simulink model "gm_sampleModel1782_4_sub"  (R2023a)
settings: Solver=VariableStepAuto  StartTime=0.0  StopTime=10.0  RelTol=1e-3
libraries: hdlsllib x1
settings Model: Creator=user1  LastModifiedBy=user1
settings OptimizationCC: BlockReduction=off  ConditionallyExecuteInputs=off
settings DebuggingCC: InheritedTsInSrcMsg=none

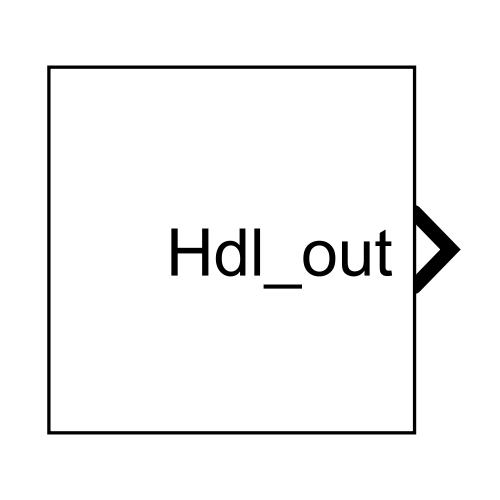
[thumbnail: Simulink's stored preview of the top-level diagram]
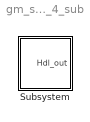
== system gm_sampleModel1782_4_sub ==
  Subsystem : Subsystem

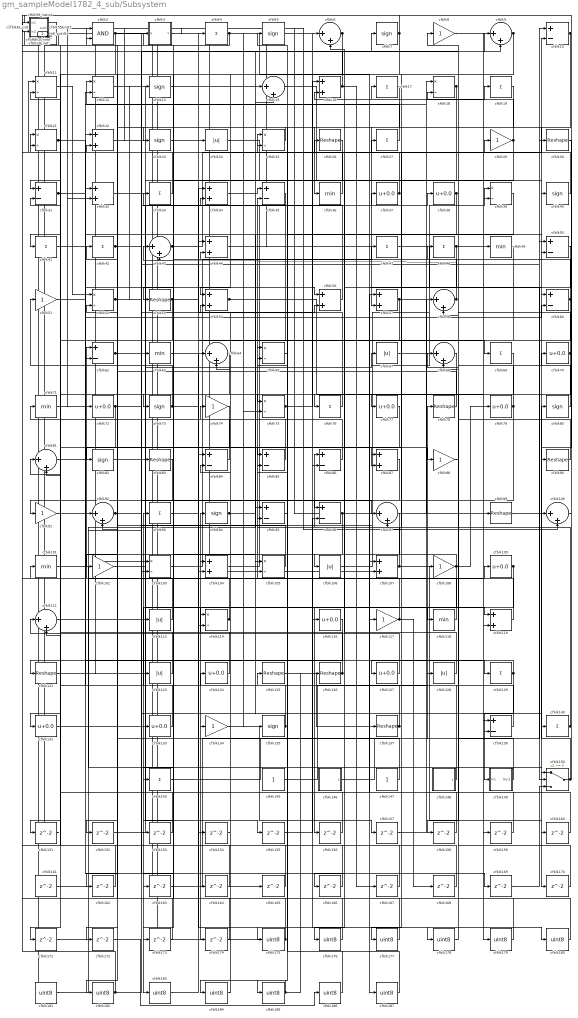
== system gm_sampleModel1782_4_sub/Subsystem ==
  cfblk1 : hdlsllib/Logic and Bit Operations/Bit Slice  lidx=7  ridx=0
  cfblk{10,31,35,50,60,62,84..86,95..96,139} (12 alike) : Sum  Inputs=+-  OutDataTypeStr=uint8
  cfblk{6,9,15,43,58,64,68,81,92,97,100,111} (12 alike) : Sum  Inputs=|++  OutDataTypeStr=uint8
  cfblk{36,49,63,71,101,118} (6 alike) : MinMax  OutDataTypeStr=uint8
  cfblk{8,29,51,74,88,91,102,108,117,134} (10 alike) : Gain  OutDataTypeStr=uint8
  cfblk{11..12,18,21,25,39,52,65,75,103,105,114} (12 alike) : Product  Inputs=*/  OutDataTypeStr=uint8  RndMeth=Zero  SaturateOnIntegerOverflow=on
  cfblk{16,22,32,34,44,54,56..57,87,104,107,119} (12 alike) : Sum  OutDataTypeStr=uint8
  cfblk{24,67,106,113,123,128} (6 alike) : Abs  OutDataTypeStr=uint8  SaturateOnIntegerOverflow=off
  cfblk{37..38,70,72,77,79,109,116,124,127,131,133} (12 alike) : Bias  Bias=0.0  SaturateOnIntegerOverflow=off
  cfblk110_inst : Subsystem
  cfblk112_inst : Subsystem
  cfblk115_inst : Subsystem
  cfblk{26,30,53,78,83,90,99,121,125..126,137} (11 alike) : Reshape
  cfblk122_inst : Subsystem
  cfblk{4,17,19,27,33,41..42,47..48,69,76,93,129,140,143} (15 alike) : Sum  Inputs=+  OutDataTypeStr=uint8
  cfblk{5,7,13,23,40,73,80,82,94,135} (10 alike) : Signum
  cfblk136_inst : Subsystem
  cfblk138_inst : Subsystem
  cfblk145 : Constant  OutDataTypeStr=uint8  SampleTime=-1
  cfblk146 : Subsystem  mask(Counter Limited){uplimit=double(7), tsamp=double(-1)}
      mask prompts: uplimit "Simulink:masks:UpperLimit_MP"; tsamp "Simulink:masks:SampleTime_MP"
      mask help: Simulink:masks:CounterLimited_MD
      mask init:
      | nbits = double(8);
      | tsamp = double(-1);
      | uplimit = double(7);
  cfblk147 : Constant  OutDataTypeStr=uint8  SampleTime=-1
  cfblk148 : Subsystem  mask(Counter Limited){uplimit=double(7), tsamp=double(-1)}
      mask prompts: uplimit "Simulink:masks:UpperLimit_MP"; tsamp "Simulink:masks:SampleTime_MP"
      mask help: Simulink:masks:CounterLimited_MD
      mask init:
      | nbits = double(8);
      | tsamp = double(-1);
      | uplimit = double(7);
  cfblk149 : Subsystem
  cfblk14_inst : Subsystem
  cfblk150 : Switch  OutDataTypeStr=uint8  SaturateOnIntegerOverflow=off  InputSameDT=off
  cfblk{151..174} (24 alike) : Delay  SampleTime=1
  cfblk{175..187} (13 alike) : DataTypeConversion  OutDataTypeStr=uint8  SaturateOnIntegerOverflow=off  RndMeth=Floor
  cfblk2 : Logic  AllPortsSameDT=off  OutDataTypeStr=boolean
  cfblk20_inst : Subsystem
  cfblk28_inst : Subsystem
  cfblk3 : Subsystem  mask(Detect Fall Nonpositive){vinit=double(0), InputProcessing=Elements as channels (sample based), OutDataTypeStr=uint8}
      mask prompts: vinit "Simulink:masks:InitialCondition_MP"; InputProcessing "Simulink:masks:InputProcessing_MP"; OutDataTypeStr "Simulink:masks:OutputDataType_MP"
      mask help: Simulink:masks:DetectFallNonpositive_MD
      mask init:
      | InputProcessing = 'Elements as channels (sample based)';
      | OutDataTypeStr = 'uint8';
      | vinit = double(0);
      mask TypeOptions InputProcessing: Simulink:masks:ColumnsAsChannelsFrameBased | Simulink:masks:ElementsAsChannelsSampleBased
      mask TypeOptions OutDataTypeStr: Simulink:masks:uint8 | Simulink:masks:boolean
      mask Display: fprintf('U <= 0\n&  NOT\nU/z <= 0')
  cfblk55_inst : Subsystem
  cfblk59_inst : Subsystem
  cfblk61_inst : Subsystem
  Hdl_out : Outport  OutDataTypeStr=uint8  SampleTime=1
  wires:
  cfblk1/1 -> cfblk61_inst/2(in2)
  cfblk10/1 -> cfblk57/2, cfblk170/1, cfblk36/1
  cfblk100/1 -> cfblk115_inst/1(in1)
  cfblk101/1 -> cfblk150/1
  cfblk102/1 -> cfblk119/1
  cfblk103/1 -> cfblk47/1
  cfblk104/1 -> cfblk37/1
  cfblk105/1 -> cfblk122_inst/2(in2)
  cfblk106/1 -> cfblk39/1
  cfblk107/1 -> cfblk35/2, cfblk160/1
  cfblk108/1 -> cfblk79/1, cfblk183/1, cfblk106/1, cfblk174/1
  cfblk109/1 -> cfblk156/1, cfblk134/1
  cfblk11/1 -> cfblk52/1
  cfblk110_inst/1(out1) -> cfblk32/2
  cfblk111/1 -> cfblk67/1
  cfblk112_inst/1(out1) -> cfblk6/1
  cfblk113/1 -> cfblk42/1
  cfblk114/1 -> cfblk62/1, cfblk138_inst/1(in1)
  cfblk115_inst/1(out1) -> cfblk24/1, cfblk14_inst/1(in1)
  cfblk116/1 -> cfblk121/1
  cfblk117/1 -> cfblk2/1, cfblk168/1
  cfblk118/1 -> cfblk95/2
  cfblk119/1 -> cfblk92/1
  cfblk12/1 -> cfblk155/1
  cfblk121/1 -> cfblk109/1
  cfblk122_inst/1(out1) -> cfblk20_inst/2(in2)
  cfblk123/1 -> cfblk28_inst/1(in1)
  cfblk124/1 -> cfblk59_inst/1(in1)
  cfblk125/1 -> cfblk137/1
  cfblk126/1 -> cfblk94/1, cfblk110_inst/2(in2)
  cfblk127/1 -> cfblk111/1
  cfblk128/1 -> cfblk6/2
  cfblk129/1 -> cfblk127/1, cfblk149/1(In1)
  cfblk13/1 -> cfblk15/1
  cfblk131/1 -> cfblk38/1
  cfblk133/1 -> cfblk101/1
  cfblk134/1 -> cfblk157/1
  cfblk135/1 -> cfblk125/1, cfblk21/1
  cfblk136_inst/1(out1) -> cfblk49/1
  cfblk137/1 -> cfblk21/2, cfblk93/1
  cfblk138_inst/1(out1) -> cfblk14_inst/2(in2), cfblk4/1
  cfblk139/1 -> cfblk74/1
  cfblk14_inst/1(out1) -> cfblk107/2, cfblk161/1
  cfblk140/1 -> cfblk86/1, cfblk27/1
  cfblk143/1 -> cfblk107/1
  cfblk145/1 -> cfblk78/1
  cfblk146/1(y) -> cfblk128/1
  cfblk147/1 -> cfblk62/2
  cfblk148/1(y) -> cfblk32/1
  cfblk149/1(Out1) -> cfblk108/1
  cfblk15/1 -> cfblk119/2
  cfblk150/1 -> cfblk80/1, cfblk70/1
  cfblk151/1 -> cfblk1/1
  cfblk152/1 -> cfblk39/2
  cfblk153/1 -> cfblk22/2
  cfblk154/1 -> cfblk84/2
  cfblk155/1 -> cfblk96/2
  cfblk156/1 -> cfblk85/2
  cfblk157/1 -> cfblk58/1
  cfblk158/1 -> cfblk81/1
  cfblk159/1 -> cfblk57/1
  cfblk16/1 -> cfblk112_inst/2(in2), cfblk167/1
  cfblk160/1 -> cfblk54/2
  cfblk161/1 -> cfblk104/1
  cfblk162/1 -> cfblk61_inst/1(in1)
  cfblk163/1 -> cfblk10/1
  cfblk164/1 -> cfblk122_inst/1(in1)
  cfblk165/1 -> cfblk11/2
  cfblk166/1 -> cfblk136_inst/2(in2)
  cfblk167/1 -> cfblk114/1
  cfblk168/1 -> cfblk43/1
  cfblk169/1 -> cfblk150/3
  cfblk17/1 -> cfblk82/1
  cfblk170/1 -> cfblk18/2
  cfblk171/1 -> cfblk15/2
  cfblk172/1 -> cfblk186/1
  cfblk173/1 -> cfblk92/2
  cfblk174/1 -> cfblk28_inst/2(in2)
  cfblk175/1 -> cfblk124/1, Hdl_out/1
  cfblk176/1 -> cfblk3/1(U)
  cfblk177/1 -> cfblk55_inst/1(in1)
  cfblk178/1 -> cfblk68/1
  cfblk179/1 -> cfblk68/2
  cfblk18/1 -> cfblk53/1, cfblk176/1
  cfblk180/1 -> cfblk55_inst/2(in2)
  cfblk181/1 -> cfblk63/1
  cfblk182/1 -> cfblk95/1, cfblk9/2, cfblk110_inst/1(in1)
  cfblk183/1 -> cfblk64/1
  cfblk184/1 -> cfblk64/2
  cfblk185/1 -> cfblk184/1, cfblk126/1
  cfblk186/1 -> cfblk65/1
  cfblk187/1 -> cfblk65/2
  cfblk19/1 -> cfblk75/1
  cfblk2/1 -> cfblk169/1, cfblk41/1
  cfblk20_inst/1(out1) -> cfblk100/2, cfblk103/1
  cfblk21/1 -> cfblk88/1, cfblk171/1, cfblk103/2
  cfblk22/1 -> cfblk40/1
  cfblk23/1 -> cfblk69/1
  cfblk24/1 -> cfblk159/1
  cfblk25/1 -> cfblk23/1
  cfblk26/1 -> cfblk73/1
  cfblk27/1 -> cfblk12/1
  cfblk28_inst/1(out1) -> cfblk72/1, cfblk100/1
  cfblk29/1 -> cfblk16/2, cfblk166/1
  cfblk3/1(Y) -> cfblk175/1
  cfblk30/1 -> cfblk90/1
  cfblk31/1 -> cfblk50/2, cfblk164/1
  cfblk32/1 -> cfblk105/1
  cfblk33/1 -> cfblk112_inst/1(in1)
  cfblk34/1 -> cfblk35/1
  cfblk35/1 -> cfblk151/1
  cfblk36/1 -> cfblk20_inst/1(in1)
  cfblk37/1 -> cfblk16/1, cfblk136_inst/1(in1)
  cfblk38/1 -> cfblk86/2, cfblk8/1
  cfblk39/1 -> cfblk85/1
  cfblk4/1 -> cfblk2/2, cfblk75/2, cfblk117/1
  cfblk40/1 -> cfblk11/1
  cfblk41/1 -> cfblk56/1
  cfblk42/1 -> cfblk87/2, cfblk105/2
  cfblk43/1 -> cfblk10/2, cfblk25/1
  cfblk44/1 -> cfblk60/1
  cfblk47/1 -> cfblk150/2
  cfblk48/1 -> cfblk44/2, cfblk76/1
  cfblk49/1 -> cfblk96/1
  cfblk5/1 -> cfblk116/1
  cfblk50/1 -> cfblk87/1
  cfblk51/1 -> cfblk12/2
  cfblk52/1 -> cfblk133/1, cfblk13/1
  cfblk53/1 -> cfblk84/1, cfblk131/1, cfblk143/1
  cfblk54/1 -> cfblk179/1, cfblk135/1
  cfblk55_inst/1(out1) -> cfblk165/1
  cfblk56/1 -> cfblk33/1
  cfblk57/1 -> cfblk99/1, cfblk114/2
  cfblk58/1 -> cfblk43/2, cfblk26/1, cfblk25/2
  cfblk59_inst/1(out1) -> cfblk83/1, cfblk181/1
  cfblk6/1 -> cfblk31/1, cfblk163/1
  cfblk60/1 -> cfblk77/1, cfblk115_inst/2(in2)
  cfblk61_inst/1(out1) -> cfblk123/1
  cfblk62/1 -> cfblk97/1, cfblk50/1, cfblk139/2
  cfblk63/1 -> cfblk180/1
  cfblk64/1 -> cfblk182/1
  cfblk65/1 -> cfblk185/1
  cfblk67/1 -> cfblk19/1
  cfblk68/1 -> cfblk177/1
  cfblk69/1 -> cfblk158/1
  cfblk7/1 -> cfblk59_inst/2(in2), cfblk54/1
  cfblk70/1 -> cfblk138_inst/2(in2), cfblk111/2
  cfblk71/1 -> cfblk129/1
  cfblk72/1 -> cfblk81/2, cfblk34/2
  cfblk73/1 -> cfblk51/1, cfblk118/1
  cfblk74/1 -> cfblk113/1
  cfblk75/1 -> cfblk178/1, cfblk29/1
  cfblk76/1 -> cfblk34/1
  cfblk77/1 -> cfblk162/1
  cfblk78/1 -> cfblk52/2
  cfblk79/1 -> cfblk44/1, cfblk102/1
  cfblk8/1 -> cfblk139/1
  cfblk80/1 -> cfblk17/1
  cfblk81/1 -> cfblk18/1
  cfblk82/1 -> cfblk56/2
  cfblk83/1 -> cfblk172/1
  cfblk84/1 -> cfblk71/1
  cfblk85/1 -> cfblk22/1
  cfblk86/1 -> cfblk31/2
  cfblk87/1 -> cfblk91/1
  cfblk88/1 -> cfblk58/2
  cfblk9/1 -> cfblk97/2, cfblk152/1
  cfblk90/1 -> cfblk48/1
  cfblk91/1 -> cfblk60/2
  cfblk92/1 -> cfblk9/1, cfblk104/2
  cfblk93/1 -> cfblk154/1
  cfblk94/1 -> cfblk7/1, cfblk140/1
  cfblk95/1 -> cfblk5/1
  cfblk96/1 -> cfblk187/1, cfblk173/1
  cfblk97/1 -> cfblk153/1
  cfblk99/1 -> cfblk30/1

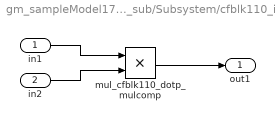
== system gm_sampleModel1782_4_sub/Subsystem/cfblk110_inst ==
  in1 : Inport  OutDataTypeStr=uint8  SampleTime=1
  in2 : Inport  Port=2  OutDataTypeStr=uint8  SampleTime=1
  mul_cfblk110_dotp_mulcomp : Product  Inputs=**  OutDataTypeStr=uint8  SampleTime=1
  out1 : Outport  OutDataTypeStr=uint8  SampleTime=1
  wires:
  in1/1 -> mul_cfblk110_dotp_mulcomp/1
  in2/1 -> mul_cfblk110_dotp_mulcomp/2
  mul_cfblk110_dotp_mulcomp/1 -> out1/1

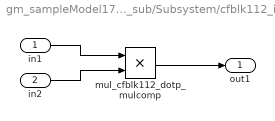
== system gm_sampleModel1782_4_sub/Subsystem/cfblk112_inst ==
  in1 : Inport  OutDataTypeStr=uint8  SampleTime=1
  in2 : Inport  Port=2  OutDataTypeStr=uint8  SampleTime=1
  mul_cfblk112_dotp_mulcomp : Product  Inputs=**  OutDataTypeStr=uint8  SampleTime=1
  out1 : Outport  OutDataTypeStr=uint8  SampleTime=1
  wires:
  in1/1 -> mul_cfblk112_dotp_mulcomp/1
  in2/1 -> mul_cfblk112_dotp_mulcomp/2
  mul_cfblk112_dotp_mulcomp/1 -> out1/1

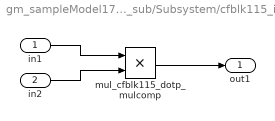
== system gm_sampleModel1782_4_sub/Subsystem/cfblk115_inst ==
  in1 : Inport  OutDataTypeStr=uint8  SampleTime=1
  in2 : Inport  Port=2  OutDataTypeStr=uint8  SampleTime=1
  mul_cfblk115_dotp_mulcomp : Product  Inputs=**  OutDataTypeStr=uint8  SampleTime=1
  out1 : Outport  OutDataTypeStr=uint8  SampleTime=1
  wires:
  in1/1 -> mul_cfblk115_dotp_mulcomp/1
  in2/1 -> mul_cfblk115_dotp_mulcomp/2
  mul_cfblk115_dotp_mulcomp/1 -> out1/1

== system gm_sampleModel1782_4_sub/Subsystem/cfblk122_inst ==
  in1 : Inport  OutDataTypeStr=uint8  SampleTime=1
  in2 : Inport  Port=2  OutDataTypeStr=uint8  SampleTime=1
  mul_cfblk122_dotp_mulcomp : Product  Inputs=**  OutDataTypeStr=uint8  SampleTime=1
  out1 : Outport  OutDataTypeStr=uint8  SampleTime=1
  wires:
  in1/1 -> mul_cfblk122_dotp_mulcomp/1
  in2/1 -> mul_cfblk122_dotp_mulcomp/2
  mul_cfblk122_dotp_mulcomp/1 -> out1/1

== system gm_sampleModel1782_4_sub/Subsystem/cfblk136_inst ==
  in1 : Inport  OutDataTypeStr=uint8  SampleTime=1
  in2 : Inport  Port=2  OutDataTypeStr=uint8  SampleTime=1
  mul_cfblk136_dotp_mulcomp : Product  Inputs=**  OutDataTypeStr=uint8  SampleTime=1
  out1 : Outport  OutDataTypeStr=uint8  SampleTime=1
  wires:
  in1/1 -> mul_cfblk136_dotp_mulcomp/1
  in2/1 -> mul_cfblk136_dotp_mulcomp/2
  mul_cfblk136_dotp_mulcomp/1 -> out1/1

== system gm_sampleModel1782_4_sub/Subsystem/cfblk138_inst ==
  in1 : Inport  OutDataTypeStr=uint8  SampleTime=1
  in2 : Inport  Port=2  OutDataTypeStr=uint8  SampleTime=1
  mul_cfblk138_dotp_mulcomp : Product  Inputs=**  OutDataTypeStr=uint8  SampleTime=1
  out1 : Outport  OutDataTypeStr=uint8  SampleTime=1
  wires:
  in1/1 -> mul_cfblk138_dotp_mulcomp/1
  in2/1 -> mul_cfblk138_dotp_mulcomp/2
  mul_cfblk138_dotp_mulcomp/1 -> out1/1

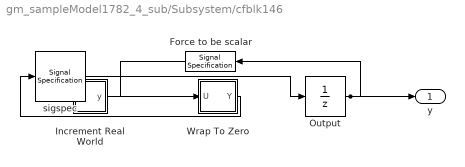
== system gm_sampleModel1782_4_sub/Subsystem/cfblk146 ==
  Force to be scalar : SignalSpecification  DisableCoverage=on  Dimensions=1
  Increment Real World : Subsystem  mask(Real World Value Increment){}
      mask help: Simulink:masks:RealWorldValueIncrement_MD
      mask Display: disp('V++')
  Output : UnitDelay  InitialCondition=0.0  SampleTime=tsamp  HasFrameUpgradeWarning=on
  Wrap To Zero : Subsystem  mask(Wrap To Zero){Threshold=double(7)}
      mask prompts: Threshold "Simulink:masks:Threshold_MP"
      mask help: Simulink:masks:WrapToZero_MD
  sigspec : SignalSpecification  OutDataTypeStr=uint8  Dimensions=1
  y : Outport  SampleTime=1
  wires:
  Force to be scalar/1 -> Increment Real World/1(u)
  Increment Real World/1(y) -> Wrap To Zero/1(U)
  Output/1 -> Force to be scalar/1, y/1
  Wrap To Zero/1(Y) -> sigspec/1
  sigspec/1 -> Output/1

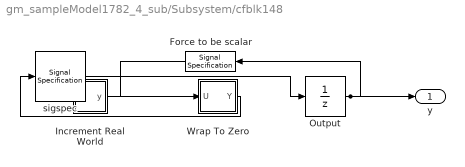
== system gm_sampleModel1782_4_sub/Subsystem/cfblk148 ==
  Force to be scalar : SignalSpecification  DisableCoverage=on  Dimensions=1
  Increment Real World : Subsystem  mask(Real World Value Increment){}
      mask help: Simulink:masks:RealWorldValueIncrement_MD
      mask Display: disp('V++')
  Output : UnitDelay  InitialCondition=0.0  SampleTime=tsamp  HasFrameUpgradeWarning=on
  Wrap To Zero : Subsystem  mask(Wrap To Zero){Threshold=double(7)}
      mask prompts: Threshold "Simulink:masks:Threshold_MP"
      mask help: Simulink:masks:WrapToZero_MD
  sigspec : SignalSpecification  OutDataTypeStr=uint8  Dimensions=1
  y : Outport  SampleTime=1
  wires:
  Force to be scalar/1 -> Increment Real World/1(u)
  Increment Real World/1(y) -> Wrap To Zero/1(U)
  Output/1 -> Force to be scalar/1, y/1
  Wrap To Zero/1(Y) -> sigspec/1
  sigspec/1 -> Output/1

== system gm_sampleModel1782_4_sub/Subsystem/cfblk149 ==
  In1 : Inport  OutDataTypeStr=uint8  PortDimensions=1  SampleTime=1
  Out1 : Outport  SampleTime=1
  wires:
  In1/1 -> Out1/1

== system gm_sampleModel1782_4_sub/Subsystem/cfblk14_inst ==
  in1 : Inport  OutDataTypeStr=uint8  SampleTime=1
  in2 : Inport  Port=2  OutDataTypeStr=uint8  SampleTime=1
  mul_cfblk14_dotp_mulcomp : Product  Inputs=**  OutDataTypeStr=uint8  SampleTime=1
  out1 : Outport  OutDataTypeStr=uint8  SampleTime=1
  wires:
  in1/1 -> mul_cfblk14_dotp_mulcomp/1
  in2/1 -> mul_cfblk14_dotp_mulcomp/2
  mul_cfblk14_dotp_mulcomp/1 -> out1/1

== system gm_sampleModel1782_4_sub/Subsystem/cfblk20_inst ==
  in1 : Inport  OutDataTypeStr=uint8  SampleTime=1
  in2 : Inport  Port=2  OutDataTypeStr=uint8  SampleTime=1
  mul_cfblk20_dotp_mulcomp : Product  Inputs=**  OutDataTypeStr=uint8  SampleTime=1
  out1 : Outport  OutDataTypeStr=uint8  SampleTime=1
  wires:
  in1/1 -> mul_cfblk20_dotp_mulcomp/1
  in2/1 -> mul_cfblk20_dotp_mulcomp/2
  mul_cfblk20_dotp_mulcomp/1 -> out1/1

== system gm_sampleModel1782_4_sub/Subsystem/cfblk28_inst ==
  in1 : Inport  OutDataTypeStr=uint8  SampleTime=1
  in2 : Inport  Port=2  OutDataTypeStr=uint8  SampleTime=1
  mul_cfblk28_dotp_mulcomp : Product  Inputs=**  OutDataTypeStr=uint8  SampleTime=1
  out1 : Outport  OutDataTypeStr=uint8  SampleTime=1
  wires:
  in1/1 -> mul_cfblk28_dotp_mulcomp/1
  in2/1 -> mul_cfblk28_dotp_mulcomp/2
  mul_cfblk28_dotp_mulcomp/1 -> out1/1

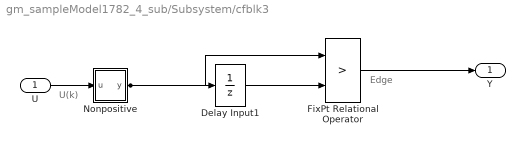
== system gm_sampleModel1782_4_sub/Subsystem/cfblk3 ==
  note: U(k)
  note: Edge
  U : Inport  OutDataTypeStr=uint8  SampleTime=1
  Delay Input1 : UnitDelay  Description=Store in Global RAM  DisableCoverage=on  InitialCondition=vinit  SampleTime=-1  HasFrameUpgradeWarning=on
  FixPt Relational Operator : RelationalOperator  Operator=>  OutDataTypeStr=fixdt(0, 8)  ZeroCross=off  InputSameDT=off
  Nonpositive : Subsystem  mask(Compare To Zero){relop=<=, OutDataTypeStr=boolean, ZeroCross=off}
      mask prompts: relop "Simulink:masks:Operator_MP"; OutDataTypeStr "Simulink:masks:OutputDataType_MP"; ZeroCross "Simulink:masks:EnableZerocrossingDetection_MP"
      mask help: Simulink:masks:CompareToZero_MD
      mask init:
      | OutDataTypeStr = 'boolean';
      | ZeroCross = 'off';
      | blkName = 'sampleModel1782_4_sub/Subsystem/cfblk3/Nonpositive';
      | relop = '<=';
      | setValue = 'boolean';
      mask TypeOptions relop: == | ~= | < | <= | >= | >
      mask TypeOptions OutDataTypeStr: Simulink:masks:uint8 | Simulink:masks:boolean
      mask Callback ZeroCross: sl('zeroCrossEnable', gcbh);
      mask Display: disp([relop,' 0'])
  Y : Outport  SampleTime=1
  wires:
  U/1 -> Nonpositive/1(u)
  Delay Input1/1 -> FixPt Relational Operator/2
  FixPt Relational Operator/1 -> Y/1
  Nonpositive/1(y) -> FixPt Relational Operator/1, Delay Input1/1

== system gm_sampleModel1782_4_sub/Subsystem/cfblk55_inst ==
  in1 : Inport  OutDataTypeStr=uint8  SampleTime=1
  in2 : Inport  Port=2  OutDataTypeStr=uint8  SampleTime=1
  mul_cfblk55_dotp_mulcomp : Product  Inputs=**  OutDataTypeStr=uint8  SampleTime=1
  out1 : Outport  OutDataTypeStr=uint8  SampleTime=1
  wires:
  in1/1 -> mul_cfblk55_dotp_mulcomp/1
  in2/1 -> mul_cfblk55_dotp_mulcomp/2
  mul_cfblk55_dotp_mulcomp/1 -> out1/1

== system gm_sampleModel1782_4_sub/Subsystem/cfblk59_inst ==
  in1 : Inport  OutDataTypeStr=uint8  SampleTime=1
  in2 : Inport  Port=2  OutDataTypeStr=uint8  SampleTime=1
  mul_cfblk59_dotp_mulcomp : Product  Inputs=**  OutDataTypeStr=uint8  SampleTime=1
  out1 : Outport  OutDataTypeStr=uint8  SampleTime=1
  wires:
  in1/1 -> mul_cfblk59_dotp_mulcomp/1
  in2/1 -> mul_cfblk59_dotp_mulcomp/2
  mul_cfblk59_dotp_mulcomp/1 -> out1/1

== system gm_sampleModel1782_4_sub/Subsystem/cfblk61_inst ==
  in1 : Inport  OutDataTypeStr=uint8  SampleTime=1
  in2 : Inport  Port=2  OutDataTypeStr=uint8  SampleTime=1
  mul_cfblk61_dotp_mulcomp : Product  Inputs=**  OutDataTypeStr=uint8  SampleTime=1
  out1 : Outport  OutDataTypeStr=uint8  SampleTime=1
  wires:
  in1/1 -> mul_cfblk61_dotp_mulcomp/1
  in2/1 -> mul_cfblk61_dotp_mulcomp/2
  mul_cfblk61_dotp_mulcomp/1 -> out1/1

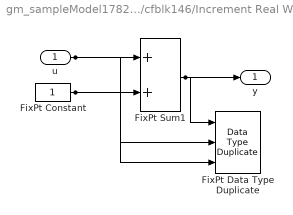
== system gm_sampleModel1782_4_sub/Subsystem/cfblk146/Increment Real World ==
  u : Inport  OutDataTypeStr=uint8  SampleTime=1
  FixPt Constant : Constant  DisableCoverage=on  OutDataTypeStr=Inherit: Inherit via back propagation  SampleTime=-1
  FixPt Data Type Duplicate : DataTypeDuplicate  DisableCoverage=on  NumInputPorts=3
  FixPt Sum1 : Sum  InputSameDT=on  OutDataTypeStr=Inherit: Inherit via back propagation  LockScale=on
  y : Outport  SampleTime=1
  wires:
  u/1 -> FixPt Sum1/1, FixPt Data Type Duplicate/2
  FixPt Constant/1 -> FixPt Sum1/2, FixPt Data Type Duplicate/3
  FixPt Sum1/1 -> FixPt Data Type Duplicate/1, y/1

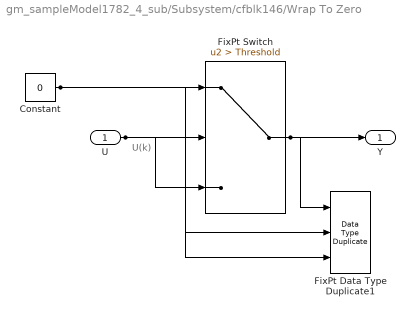
== system gm_sampleModel1782_4_sub/Subsystem/cfblk146/Wrap To Zero ==
  note: U(k)
  U : Inport  OutDataTypeStr=uint8  SampleTime=1
  Constant : Constant  DisableCoverage=on  Value=0  OutDataTypeStr=Inherit: Inherit via back propagation  SampleTime=-1
  FixPt Data Type Duplicate1 : DataTypeDuplicate  DisableCoverage=on  NumInputPorts=3
  FixPt Switch : Switch  Criteria=u2 > Threshold  Threshold=Threshold  OutDataTypeStr=Inherit: Inherit via back propagation  ZeroCross=off  SaturateOnIntegerOverflow=off  InputSameDT=off
  Y : Outport  SampleTime=1
  wires:
  U/1 -> FixPt Switch/3, FixPt Switch/2, FixPt Data Type Duplicate1/2
  Constant/1 -> FixPt Switch/1, FixPt Data Type Duplicate1/3
  FixPt Switch/1 -> FixPt Data Type Duplicate1/1, Y/1

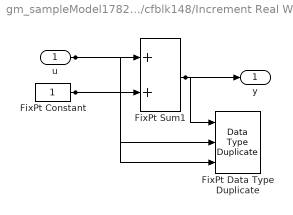
== system gm_sampleModel1782_4_sub/Subsystem/cfblk148/Increment Real World ==
  u : Inport  OutDataTypeStr=uint8  SampleTime=1
  FixPt Constant : Constant  DisableCoverage=on  OutDataTypeStr=Inherit: Inherit via back propagation  SampleTime=-1
  FixPt Data Type Duplicate : DataTypeDuplicate  DisableCoverage=on  NumInputPorts=3
  FixPt Sum1 : Sum  InputSameDT=on  OutDataTypeStr=Inherit: Inherit via back propagation  LockScale=on
  y : Outport  SampleTime=1
  wires:
  u/1 -> FixPt Sum1/1, FixPt Data Type Duplicate/2
  FixPt Constant/1 -> FixPt Sum1/2, FixPt Data Type Duplicate/3
  FixPt Sum1/1 -> FixPt Data Type Duplicate/1, y/1

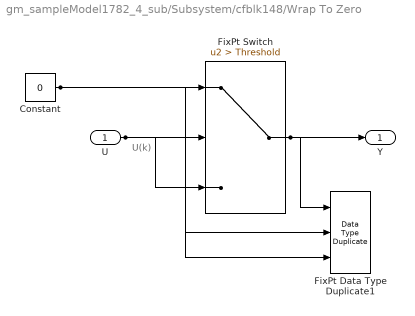
== system gm_sampleModel1782_4_sub/Subsystem/cfblk148/Wrap To Zero ==
  note: U(k)
  U : Inport  OutDataTypeStr=uint8  SampleTime=1
  Constant : Constant  DisableCoverage=on  Value=0  OutDataTypeStr=Inherit: Inherit via back propagation  SampleTime=-1
  FixPt Data Type Duplicate1 : DataTypeDuplicate  DisableCoverage=on  NumInputPorts=3
  FixPt Switch : Switch  Criteria=u2 > Threshold  Threshold=Threshold  OutDataTypeStr=Inherit: Inherit via back propagation  ZeroCross=off  SaturateOnIntegerOverflow=off  InputSameDT=off
  Y : Outport  SampleTime=1
  wires:
  U/1 -> FixPt Switch/3, FixPt Switch/2, FixPt Data Type Duplicate1/2
  Constant/1 -> FixPt Switch/1, FixPt Data Type Duplicate1/3
  FixPt Switch/1 -> FixPt Data Type Duplicate1/1, Y/1

== system gm_sampleModel1782_4_sub/Subsystem/cfblk3/Nonpositive ==
  u : Inport  OutDataTypeStr=uint8  SampleTime=1
  Compare : RelationalOperator  Operator=<=  OutDataTypeStr=boolean  ZeroCross=off
  Constant : Constant  DisableCoverage=on  Value=0  OutDataTypeStr=Inherit: Inherit via back propagation  SampleTime=-1  PreserveConstantTs=on
  y : Outport  SampleTime=1
  wires:
  u/1 -> Compare/1
  Compare/1 -> y/1
  Constant/1 -> Compare/2
